simulink model "AHRS_PF"  (R2023b)
settings: Solver=ode4  StartTime=0.0  StopTime=50  FixedStep=0.01  RelTol=1e-3
libraries: simulink x1
settings Model: Creator=Alireza Sharifi  LastModifiedBy=Ali
settings OptimizationCC: ReuseModelBlockBuffer=off
settings ModelReferenceCC: EnableRefExpFcnMdlSchedulingChecks=on

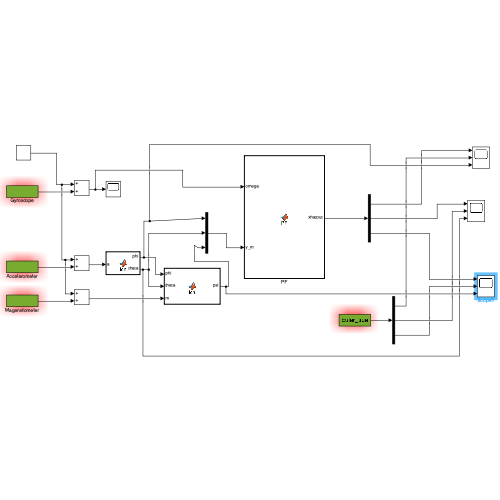
[thumbnail: Simulink's stored preview of the top-level diagram]
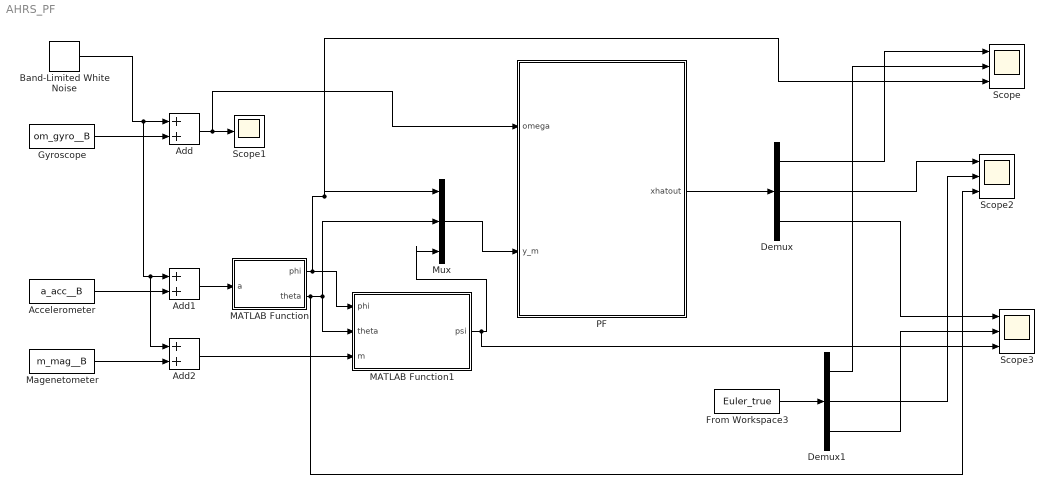
== system AHRS_PF ==
  Accelerometer : FromWorkspace  VariableName=a_acc__B  SampleTime=0.01
  Add : Sum
  Add1 : Sum
  Add2 : Sum
  Band-Limited White Noise : simulink/Sources/Band-Limited White Noise  Cov=1e-5  Ts=0.01  seed=[23341]
  Demux : Demux  Outputs=3
  Demux1 : Demux  Outputs=3
  From Workspace3 : FromWorkspace  VariableName=Euler_true  SampleTime=0.01
  Gyroscope : FromWorkspace  VariableName=om_gyro__B  SampleTime=0.01
  MATLAB Function : MATLAB Function  TreatAsAtomicUnit=on
  MATLAB Function1 : MATLAB Function  TreatAsAtomicUnit=on
  Magenetometer : FromWorkspace  VariableName=m_mag__B  SampleTime=0.01
  Mux : Mux  Inputs=3
  PF : MATLAB Function  TreatAsAtomicUnit=on
  Scope : Scope  NumInputPorts=3
  Scope1 : Scope
  Scope2 : Scope  NumInputPorts=3
  Scope3 : Scope  NumInputPorts=3
  wires:
  Gyroscope/1 -> Add/2
  Add/1 -> PF/1(omega), Scope1/1
  Accelerometer/1 -> Add1/2
  Magenetometer/1 -> Add2/2
  Band-Limited White Noise/1 -> Add2/1, Add1/1, Add/1
  Add1/1 -> MATLAB Function/1(a)
  Add2/1 -> MATLAB Function1/3(m)
  MATLAB Function/2(theta) -> Scope2/3, MATLAB Function1/2(theta), Mux/2
  MATLAB Function/1(phi) -> Scope/3, Mux/1, MATLAB Function1/1(phi)
  Mux/1 -> PF/2(y_m)
  MATLAB Function1/1(psi) -> Scope3/3, Mux/3
  PF/1(xhatout) -> Demux/1
  From Workspace3/1 -> Demux1/1
  Demux/1 -> Scope/1
  Demux/2 -> Scope2/1
  Demux/3 -> Scope3/1
  Demux1/1 -> Scope/2
  Demux1/2 -> Scope2/2
  Demux1/3 -> Scope3/2

== matlab function AHRS_PF/MATLAB Function1 ==
  data: phi input; psi output; theta input; m input
function psi = fcn(phi,theta,m)
mx=m(1);
my=m(2);
mz=m(3);
%
num_psi=-cos(phi)*my+sin(phi)*mz;
den_psi=cos(theta)*mx+sin(theta)*sin(phi)*my+sin(theta)*cos(phi)*mz;
declination_angle=-4.0266*pi/180;
psi=atan2(num_psi,den_psi)+declination_angle;

== matlab function AHRS_PF/MATLAB Function ==
  data: a input; phi output; theta output
function [phi,theta] = fcn(a)
ax=a(1);
ay=a(2);
az=a(3);
g=9.81;
phi=atan2(-ay,-az);
theta=asin(ax/g);

== matlab function AHRS_PF/PF ==
  data: omega input; xhatout output; y_m input
function xhatout = PF(omega,y_m)

%% constant parameters
N=1000;
Ts=0.01;
%% omega
p=omega(1);
q=omega(2);
r=omega(3);
%%
persistent x_hat P xpart
if isempty(x_hat)
    x_hat=[0;0;0];
end

if isempty(P)
    P=1e-5*eye(3);
end

if isempty(xpart)
    xpart = zeros(3,N); 
    P_d = [P(1,1);P(2,2);P(3,3)];
    for i = 1 : N
        xpart(:,i) = x_hat + sqrt(P_d) * randn;
    end
end

%%

Q=  0.00001*eye(3);
R=0.01*eye(3);

%% Particle filter
q_PF = zeros(N,1);
xpartminus = zeros(3,N);
for i = 1 : N
    xpartminus(1,i)=xpart(1,i)+Ts*(p+tan(xpart(2,i))*sin(xpart(1,i))*q+r*cos(xpart(1,i))*tan(xpart(2,i)))+ sqrt(Q(1,1)) * randn;
    xpartminus(2,i)=xpart(2,i)+Ts*(q*cos(xpart(1,i))-r*sin(xpart(1,i)))+ sqrt(Q(2,2)) * randn;
    xpartminus(3,i)=xpart(3,i)+Ts*(sec(xpart(2,i))*(q*sin(xpart(1,i))+r*cos(xpart(1,i)))) + sqrt(Q(3,3)) * randn;

    ypart = [xpartminus(1,i);xpartminus(2,i);xpartminus(3,i)];
    vhat = y_m - ypart;
    q_PF(i) = (1 / sqrt(det(R)) / sqrt((2*pi)^3)) * exp(-1/2*vhat'*inv(R)*vhat);

end

%% Normalize the likelihood of each a priori estimate.
    qsum = sum(q_PF);
    for i = 1 : N
        q_PF(i) = q_PF(i) / qsum;
    end

 %% Resample.
    for i = 1 : N
        u = rand; % uniform random number between 0 and 1
        qtempsum = 0;
        for j = 1 : N
            qtempsum = qtempsum + q_PF(j);
            if qtempsum >= u
                xpart(:,i) = xpartminus(:,j);
                break;
            end
        end
    end

%% The particle filter estimate is the mean of the particles.
x_hat = mean(xpart,2);
xhatout = x_hat;





% %%
% xhat1=xhat(1)+Ts*(p+tan(xhat(2))*sin(xhat(1))*q+r*cos(xhat(1))*tan(xhat(2)));
% xhat2=xhat(2)+Ts*(q*cos(xhat(1))-r*sin(xhat(1)));
% xhat3=xhat(3)+Ts*(sec(xhat(2))*(q*sin(xhat(1))+r*cos(xhat(1))));
% %%
% xhat=[xhat1;xhat2;xhat3];
% %%
% F=[1+Ts*tan(xhat(2))*(q*cos(xhat(1))-r*sin(xhat(1))) ...
%     Ts*(q*sin(xhat(1))+r*cos(xhat(1)))/(cos(xhat(2))^2) 0;
%   Ts*(-q*sin(xhat(1))-r*cos(xhat(1)))   1   0;
%   Ts*(q*cos(xhat(1))-r*sin(xhat(1)))/cos(xhat(2)) ...
%      Ts*sin(xhat(2))*(q*sin(xhat(1))+r*cos(xhat(1)))/(cos(xhat(2))^2) 1];
% Gama=[Ts Ts*tan(xhat(2))*sin(xhat(1)) Ts*tan(xhat(2))*cos(xhat(1));
%     0  Ts*cos(xhat(1))  -Ts*sin(xhat(1));
%     0  Ts*sin(xhat(1))/cos(xhat(2)) Ts*cos(xhat(1))/cos(xhat(2))];
% P=F*P*F'+Gama*Q*Gama';
% %%
% C=[1 0 0;
%     0 1 0;
%     0 0 1];
% yhat=C*xhat;
% K=P*C'*inv(C*P*C'+R);
% xhat=xhat+K*(ym-yhat);
% P=(eye(3)-K*C)*P*(eye(3)-K*C)'+K*R*K';
% xhatout=xhat;
